simulink model "motorresponse"  (R2013b)
settings: Solver=FixedStepDiscrete  SolverMode=SingleTasking  StartTime=0.0  StopTime=inf  RelTol=1e-3
undefined symbols (not defined in the file or in its folder): DiscIntNeverNeededParam
libraries: arduinolib x8, simulink x4
settings Model: SimulationMode=external  ExtModeTrigDuration=2  Creator=Joshua  LastModifiedBy=Joshua
settings OptimizationCC: OptimizeModelRefInitCode=on  LifeSpan=1
settings DebuggingCC: SolverPrmCheckMsg=none
settings HardwareCC: ProdBitPerInt=16  ProdBitPerPointer=8  ProdIntDivRoundTo=Zero  ProdEndianess=LittleEndian  ProdWordSize=8  ProdHWDeviceType=Atmel->AVR
settings RTWCC: SystemTargetFile=realtime.tlc  GenerateMakefile=off  TemplateMakefile=realtime.tmf  Description=Run on Target Hardware  RTWVerbose=off  ProcessScript=realtime_make_rtw_hook
settings STFCustomTargetCC: TargetLibSuffix=.a  GenerateSampleERTMain=on  ERTCustomFileBanners=on  SupportNonInlinedSFcns=off  SupportVariableSizeSignals=on  MATLABClassNameForMDSCustomization=Simulink.SoftwareTarget.ERTCustomization  GRTInterface=off  SystemTargetFile=realtime.tlc
settings ERTTargetCC: CodeReplacementLibrary=ANSI_C  GenerateSampleERTMain=on  ParMdlRefBuildCompliant=off  CompOptLevelCompliant=off  ConcurrentExecutionCompliant=off  CombineOutputUpdateFcns=off  ERTFirstTimeCompliant=off  SupportContinuousTime=on  SupportVariableSizeSignals=on  ModelStepFunctionPrototypeControlCompliant=off  CPPClassGenCompliant=off  ExtModeTransport=3  ExtModeMexFile=ext_serial_win32_comm  ExtModeMexArgs=0 1 9600  InlinedParameterPlacement=NonHierarchical  ERTSrcFileBannerTemplate=realtime_code_template.cgt  ERTHdrFileBannerTemplate=realtime_code_template.cgt  ERTDataSrcFileTemplate=realtime_code_template.cgt  ERTDataHdrFileTemplate=realtime_code_template.cgt  ERTCustomFileTemplate=realtime_file_process.tlc

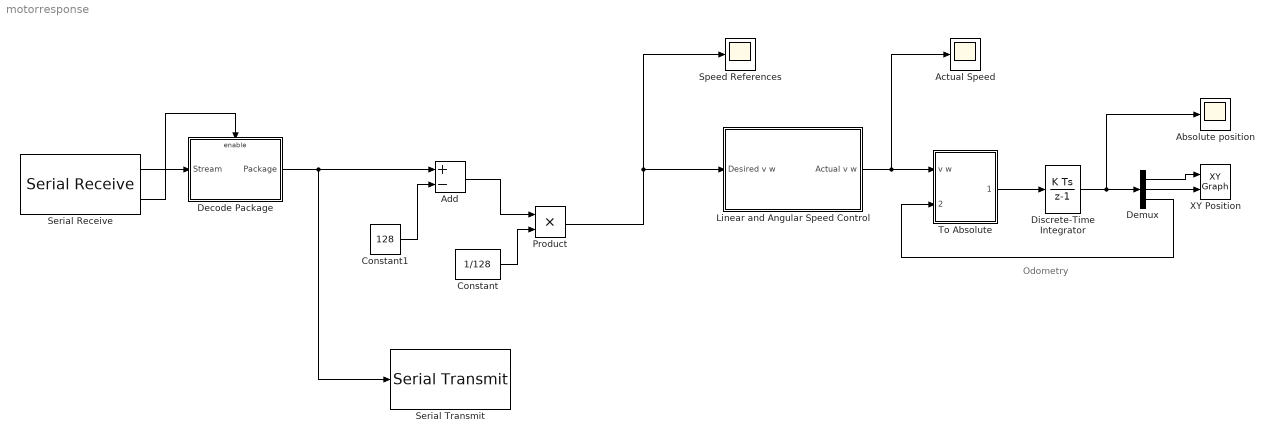
== system motorresponse ==
  note: Odometry
  Absolute position : Scope
      settings: YMin=34.7  YMax=36
  Actual Speed : Scope
      settings: YMin=34.7  YMax=36
  Add : Sum  Inputs=+-  OutDataTypeStr=double
  Constant : Constant  Value=1/128
  Constant1 : Constant  Value=128
  Decode Package : Subsystem
  Demux : Demux  Outputs=3
  Discrete-Time Integrator : DiscreteIntegrator  SampleTime=-1  ICPrevOutput=DiscIntNeverNeededParam  ICPrevScaledInput=DiscIntNeverNeededParam
  Linear and Angular Speed Control : Subsystem
  Product : Product
  Serial Receive : arduinolib/Serial Receive  portNumber=0  showOutStatus=on  sampleTime=-1
  Serial Transmit : arduinolib/Serial Transmit  portNumber=0
  Speed References : Scope
      settings: YMin=34.7  YMax=36  SaveName=ScopeData2
  To Absolute : Subsystem
  XY Position : simulink/Sinks/XY Graph  xmin=-100  xmax=100  ymin=-100  ymax=100  st=-1
  wires:
  To Absolute/1(vx vy w) -> Discrete-Time Integrator/1
  Demux/1 -> XY Position/1
  Demux/2 -> XY Position/2
  Demux/3 -> To Absolute/2(Angle)
  Discrete-Time Integrator/1 -> Absolute position/1, Demux/1
  Linear and Angular Speed Control/1(Actual v w) -> To Absolute/1(v w), Actual Speed/1
  Serial Receive/1 -> Decode Package/1(Stream)
  Serial Receive/2 -> Decode Package/Enable
  Add/1 -> Product/1
  Decode Package/1(Package) -> Serial Transmit/1, Add/1
  Constant/1 -> Product/2
  Constant1/1 -> Add/2
  Product/1 -> Speed References/1, Linear and Angular Speed Control/1(Desired v w)

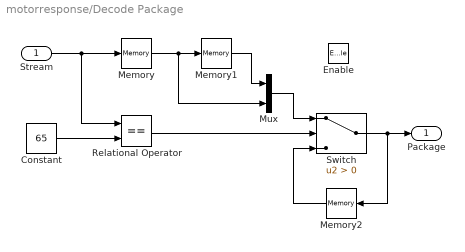
== system motorresponse/Decode Package ==
  Stream : Inport
  Enable : EnablePort
  Constant : Constant  Value=65
  Memory : Memory
  Memory1 : Memory
  Memory2 : Memory
  Mux : Mux  Inputs=2
  Relational Operator : RelationalOperator  Operator===  OutDataTypeStr=boolean
  Switch : Switch  Criteria=u2 > Threshold
  Package : Outport
  wires:
  Stream/1 -> Relational Operator/1, Memory/1
  Memory/1 -> Mux/2, Memory1/1
  Memory1/1 -> Mux/1
  Mux/1 -> Switch/1
  Relational Operator/1 -> Switch/2
  Constant/1 -> Relational Operator/2
  Switch/1 -> Memory2/1, Package/1
  Memory2/1 -> Switch/3

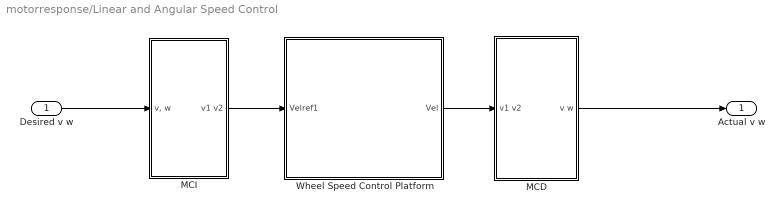
== system motorresponse/Linear and Angular Speed Control ==
  Desired v w : Inport
  MCD : Subsystem
  MCI : Subsystem  mask{d=0.22}
      mask prompts: d "Distancia entre ruedas"
  Wheel Speed Control Platform : Subsystem
      mask Display: image('imagen_robot.png')
  Actual v w : Outport
  wires:
  Desired v w/1 -> MCI/1("v, w")
  MCI/1(v1 v2) -> Wheel Speed Control Platform/1(Velref1)
  MCD/1(v w) -> Actual v w/1
  Wheel Speed Control Platform/1(Vel) -> MCD/1(v1 v2)

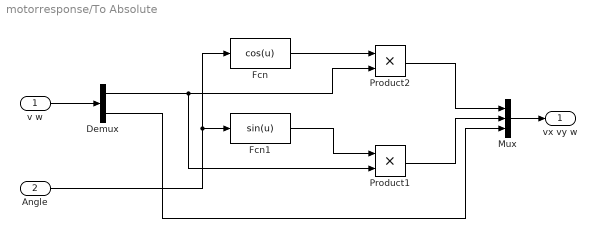
== system motorresponse/To Absolute ==
  v w : Inport
  Angle : Inport  Port=2
  Demux : Demux  Outputs=2
  Fcn : Fcn  Expr=cos(u)
  Fcn1 : Fcn  Expr=sin(u)
  Mux : Mux  Inputs=3
  Product1 : Product
  Product2 : Product
  vx vy w : Outport
  wires:
  Angle/1 -> Fcn1/1, Fcn/1
  v w/1 -> Demux/1
  Demux/2 -> Mux/3
  Mux/1 -> vx vy w/1
  Product2/1 -> Mux/1
  Product1/1 -> Mux/2
  Fcn1/1 -> Product1/1
  Demux/1 -> Product2/2, Product1/2
  Fcn/1 -> Product2/1

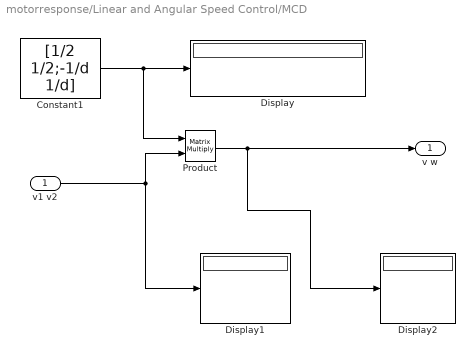
== system motorresponse/Linear and Angular Speed Control/MCD ==
  v1 v2 : Inport
  Constant1 : Constant  Value=[1/2 1/2;-1/d 1/d]  VectorParams1D=off  mask{d=0.22}
      mask prompts: d "distancia"
  Display : Display
  Display1 : Display
  Display2 : Display
  Product : Product  Multiplication=Matrix(*)
  v w : Outport
  wires:
  Product/1 -> Display2/1, v w/1
  Constant1/1 -> Display/1, Product/1
  v1 v2/1 -> Display1/1, Product/2

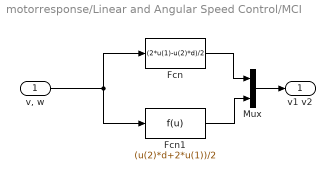
== system motorresponse/Linear and Angular Speed Control/MCI ==
  "v, w" : Inport
  Fcn : Fcn  Expr=(2*u(1)-u(2)*d)/2
  Fcn1 : Fcn  Expr=(u(2)*d+2*u(1))/2
  Mux : Mux  Inputs=2
  v1 v2 : Outport
  wires:
  Mux/1 -> v1 v2/1
  "v, w"/1 -> Fcn1/1, Fcn/1
  Fcn1/1 -> Mux/2
  Fcn/1 -> Mux/1

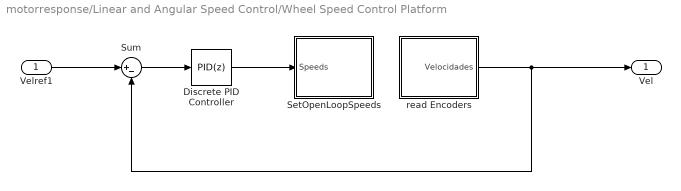
== system motorresponse/Linear and Angular Speed Control/Wheel Speed Control Platform ==
  Velref1 : Inport
  Discrete PID Controller : simulink/Continuous/PID Controller  Controller=PID  TimeDomain=Discrete-time  SampleTime=-1  IntegratorMethod=Forward Euler  FilterMethod=Forward Euler  Form=Parallel  P=1  I=2  D=0  N=100  InitialConditionSource=internal  InitialConditionForIntegrator=0  InitialConditionForFilter=0  ExternalReset=none  LimitOutput=on  UpperSaturationLimit=0.8  LowerSaturationLimit=-0.8  LinearizeAsGain=off  AntiWindupMode=clamping  Kb=1  TrackingMode=off  Kt=1  PParamMin=[]  PParamMax=[]  IParamMin=[]  IParamMax=[]  DParamMin=[]  DParamMax=[]  NParamMin=[]  NParamMax=[]  KbParamMin=[]  KbParamMax=[]  KtParamMin=[]  KtParamMax=[]  POutMin=[]  POutMax=[]  IOutMin=[]  IOutMax=[]  DOutMin=[]  DOutMax=[]  NOutMin=[]  NOutMax=[]  KbOutMin=[]  KbOutMax=[]  KtOutMin=[]  KtOutMax=[]  IntegratorOutMin=[]  IntegratorOutMax=[]  FilterOutMin=[]  FilterOutMax=[]  SumOutMin=[]  SumOutMax=[]  SumI1OutMin=[]  SumI1OutMax=[]  SumI2OutMin=[]  SumI2OutMax=[]  SumI3OutMin=[]  SumI3OutMax=[]  SumDOutMin=[]  SumDOutMax=[]  SaturationOutMin=[]  SaturationOutMax=[]  IntegratorContinuousStateAttributes=''  IntegratorStateMustResolveToSignalObject=off  IntegratorRTWStateStorageClass=Auto  FilterContinuousStateAttributes=''  FilterStateMustResolveToSignalObject=off  FilterRTWStateStorageClass=Auto
  SetOpenLoopSpeeds : Subsystem
  Sum : Sum  Inputs=|+-
  read Encoders : Subsystem
  Vel : Outport
  wires:
  read Encoders/1(Velocidades) -> Sum/2, Vel/1
  Sum/1 -> Discrete PID Controller/1
  Velref1/1 -> Sum/1
  Discrete PID Controller/1 -> SetOpenLoopSpeeds/1(Speeds)

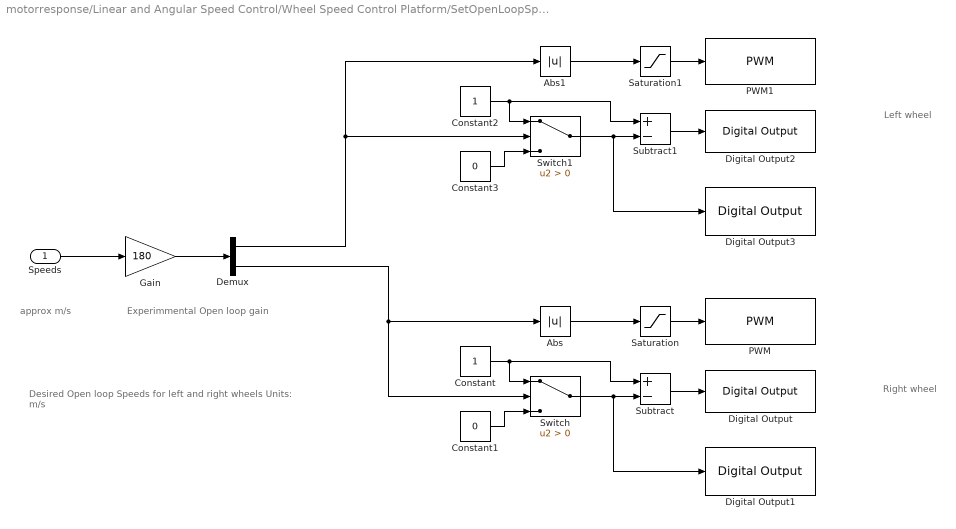
== system motorresponse/Linear and Angular Speed Control/Wheel Speed Control Platform/SetOpenLoopSpeeds ==
  note: Desired Open loop Speeds for left and right wheels
      | Units: m/s
  note: Experimmental
      | Open loop gain
  note: approx m/s
  note: Left wheel
  note: Right wheel
  Speeds : Inport
  Abs : Abs
  Abs1 : Abs
  Constant : Constant
  Constant1 : Constant  Value=0
  Constant2 : Constant
  Constant3 : Constant  Value=0
  Demux : Demux  Outputs=2
  Digital Output : arduinolib/Digital Output  pinNumber=11
  Digital Output1 : arduinolib/Digital Output  pinNumber=12
  Digital Output2 : arduinolib/Digital Output  pinNumber=9
  Digital Output3 : arduinolib/Digital Output  pinNumber=10
  Gain : Gain  Gain=180
  PWM : arduinolib/PWM  pinNumber=13
  PWM1 : arduinolib/PWM  pinNumber=8
  Saturation : Saturate  UpperLimit=255  LowerLimit=0  OutDataTypeStr=uint8
  Saturation1 : Saturate  UpperLimit=255  LowerLimit=0  OutDataTypeStr=uint8
  Subtract : Sum  Inputs=+-
  Subtract1 : Sum  Inputs=+-
  Switch : Switch  Criteria=u2 > Threshold
  Switch1 : Switch  Criteria=u2 > Threshold
  wires:
  Demux/2 -> Abs/1, Switch/2
  Demux/1 -> Abs1/1, Switch1/2
  Saturation1/1 -> PWM1/1
  Subtract1/1 -> Digital Output2/1
  Switch1/1 -> Digital Output3/1, Subtract1/2
  Constant3/1 -> Switch1/3
  Constant2/1 -> Subtract1/1, Switch1/1
  Abs1/1 -> Saturation1/1
  Saturation/1 -> PWM/1
  Subtract/1 -> Digital Output/1
  Switch/1 -> Subtract/2, Digital Output1/1
  Constant1/1 -> Switch/3
  Constant/1 -> Switch/1, Subtract/1
  Gain/1 -> Demux/1
  Abs/1 -> Saturation/1
  Speeds/1 -> Gain/1

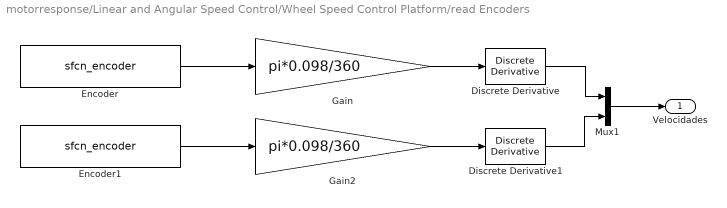
== system motorresponse/Linear and Angular Speed Control/Wheel Speed Control Platform/read Encoders ==
  Discrete Derivative : simulink/Discrete/Discrete Derivative  gainval=1.0  ICPrevScaledInput=0.0  InputProcessing=Inherited  OutMin=[]  OutMax=[]  OutDataType=fixdt(1, 16)  OutScaling=2^-10  DoSatur=off
  Discrete Derivative1 : simulink/Discrete/Discrete Derivative  gainval=1.0  ICPrevScaledInput=0.0  InputProcessing=Inherited  OutMin=[]  OutMax=[]  OutDataType=fixdt(1, 16)  OutScaling=2^-10  DoSatur=off
  Encoder : S-Function  InitFcn=try, set_param(gcb,'FunctionName','sfcn_encoder'), end  FunctionName=sfcn_encoder  Parameters=uint8(0),uint8(3),uint8(2)  SFunctionModules=sfcn_encoder_wrapper  EnableBusSupport=off  mask(S-Function Builder){}
      mask init:
      | val = [[.9  0.75 0.75 1 1 .9 .9 1]',[1 1 0.75 0.75 .9 .9 1 .9]'];try , sys = get_param(gcb,'SfunBuilderFcnName');if isempty(sys), sys = get_param(gcb,'FunctionName'); end,catch, sys = get_param(gcb,'FunctionName'); end
      settings: CopyFcn=set_param(gcbh,'LinkStatus','none')  PreSaveFcn=try, set_param(gcb,'FunctionName','sfcn_encoder'), end  OpenFcn=sfunctionwizard(gcbh)
      mask Display: plot(val(:,1),val(:,2)),disp(sys), port_label('output',1,'pos')
  Encoder1 : S-Function  InitFcn=try, set_param(gcb,'FunctionName','sfcn_encoder'), end  FunctionName=sfcn_encoder  Parameters=uint8(1),uint8(19),uint8(18)  SFunctionModules=sfcn_encoder_wrapper  EnableBusSupport=off  mask(S-Function Builder){}
      mask init: same as motorresponse/Linear and Angular Speed Control/Wheel Speed Control Platform/read Encoders/Encoder
      settings: CopyFcn=set_param(gcbh,'LinkStatus','none')  PreSaveFcn=try, set_param(gcb,'FunctionName','sfcn_encoder'), end  OpenFcn=sfunctionwizard(gcbh)
      mask Display: plot(val(:,1),val(:,2)),disp(sys), port_label('output',1,'pos')
  Gain : Gain  Gain=pi*0.098/360  OutDataTypeStr=double
  Gain2 : Gain  Gain=pi*0.098/360  OutDataTypeStr=double
  Mux1 : Mux  Inputs=2
  Velocidades : Outport
  wires:
  Mux1/1 -> Velocidades/1
  Discrete Derivative/1 -> Mux1/1
  Discrete Derivative1/1 -> Mux1/2
  Encoder1/1 -> Gain2/1
  Encoder/1 -> Gain/1
  Gain/1 -> Discrete Derivative/1
  Gain2/1 -> Discrete Derivative1/1
